simulink model "dqn_C_PQ_HVsMC"  (R2024a)
settings: Solver=FixedStepDiscrete  StartTime=0.0  StopTime=10  FixedStep=Ts_Power  RelTol=1e-3
PreLoadFcn:
  | % HVDCMMCInterconnectionParam
StartFcn:
  | tic
StopFcn:
  | toc
values from neighbouring files (symbols this model uses):
  C_PM = 1.758e-3    (= 0.001758)    [dqnMMCsingle.m]
  Fnom = 50    [dqnMMCsingle.m]
  HRM = 1    [dqnMMCsingle.m]
  Ki_Ireg = 6    [dqnMMCsingle.m]
  Ki_Qreg = 1.0    (= 1)    [dqnMMCsingle.m]
  Kp_Ireg = 0.6    [dqnMMCsingle.m]
  Kp_Qreg = 0.5/3    (= 0.166666666667)    [dqnMMCsingle.m]
  Larm = Larm_pu*(Zb_ac/(2*pi*Fnom))    [dqnMMCsingle.m]
  Larm_pu = 0.15    [dqnMMCsingle.m]
  Lff = Larm_pu/2    (= 0.075)    [dqnMMCsingle.m]
  Limits_Ireg = [ 2.0  -2.0]    [dqnMMCsingle.m]
  Limits_Qreg = [ 0.25, -0.25 ]    [dqnMMCsingle.m]
  Limits_VDCreg = [ 2.0  -2.0]    [dqnMMCsingle.m]
  Lxfo = 0.12    [dqnMMCsingle.m]
  N = 1    [dqnMMCsingle.m]
  Nb_PM = 36    [dqnMMCsingle.m]
  Pnom = 1000e6    (= 1000000000)    [dqnMMCsingle.m]
  R_startup = 400    [dqnMMCsingle.m]
  Rarm = Rarm_pu*Zb_ac    [dqnMMCsingle.m]
  Rff = Rarm_pu/2    (= 0.00075)    [dqnMMCsingle.m]
  Rxfo = 0.003    [dqnMMCsingle.m]
  Slope_Qref = 0.5    [dqnMMCsingle.m]
  Slope_Vdc_ref = Vnom_dc/5    (= 128000)    [dqnMMCsingle.m]
  Tfault = 9999    [dqnMMCsingle.m]
  Ts = Ts_Control    (= 4e-05)    [dqnMMCsingle.m]
  Ts_Control = 40e-6    (= 4e-05)    [dqnMMCsingle.m]
  Ts_dqn = 2e-5    (= 2e-05)    [dqnMMCsingle.m]
  Ts_Power = 20e-6    (= 2e-05)    [dqnMMCsingle.m]
  Vnom_dc = 640e3    (= 640000)    [dqnMMCsingle.m]
  Vnom_prim = 400e3    (= 400000)    [dqnMMCsingle.m]
  Vnom_sec = 333e3    (= 333000)    [dqnMMCsingle.m]
  Ws = 2*pi*50    (= 314.159265359)    [dqnMMCsingle.m]
undefined symbols (not defined in the file or in its folder): DiscIntNeverNeededParam, Discrete, DQN_Lib, gcbh, Int_DQNc_Mat, Mult_DQNc_Mat, Pcc, S, sps, sps_rtmsupport, spsMeanValueVariableFrequencyModel, spsPLL3phModel, SY3
libraries: simulink x18, spsControlledVoltageSourceLib x15, spsVoltageMeasurementLib x9, powerlib_extras x6, spsSecondOrderFilterLib x6, spsCurrentMeasurementLib x6, spsIdealSwitchLib x6, spsMeanLib x4, spsdq0toabcLib x4, spsMeanVariableFrequencyLib x4, spsabctodq0Lib x4, spsThreePhaseSeriesRLCBranchLib x4
(part 1 of 6)
settings Model: SimulationMode=accelerator  Creator=The MathWorks, Inc.  LastModifiedBy=salsarayreh
settings SolverCC: AlgebraicLoopSolver=TrustRegion
settings DataIOCC: SaveFormat=StructureWithTime  SaveOutput=off  DSMLogging=off  SaveTime=off  ReturnWorkspaceOutputs=off
settings OptimizationCC: ReuseModelBlockBuffer=off  ExpressionDepthLimit=2147483647  LifeSpan=inf
settings DebuggingCC: UnderspecifiedInitializationDetection=Classic  MergeDetectMultiDrivingBlocksExec=none  SolverPrmCheckMsg=warning  FcnCallInpInsideContextMsg=warning  UnconnectedInputMsg=warning  UnconnectedOutputMsg=warning  UnconnectedLineMsg=warning  AllowSymbolicDim=off  StateNameClashWarn=warning  SFUnexpectedBacktrackingDiag=warning  SFNoUnconditionalDefaultTransitionDiag=warning  SFExecutionAtInitializationDiag=none  ArithmeticOperatorsInVariantConditions=warning
settings HardwareCC: ProdBitPerPointer=32  ProdBitPerSizeT=32  ProdBitPerPtrDiffT=32  ProdLargestAtomicFloat=None  ProdIntDivRoundTo=Undefined  ProdEndianess=Unspecified  ProdWordSize=32  ProdHWDeviceType=32-bit Generic
settings ModelReferenceCC: EnableRefExpFcnMdlSchedulingChecks=on  PropagateSignalLabelsOutOfModel=off
settings SFSimCC: SimUseLocalCustomCode=off  CustomCodeUndefinedFunction=UseInterfaceOnly
settings RTWCC: RTWUseLocalCustomCode=off  GPUComputeCapability=3.5
settings CodeAppCC: StateflowObjectComments=on
settings GRTTargetCC: TargetLangStandard=C89/C90 (ANSI)  CombineOutputUpdateFcns=off  GRTInterface=on
settings ConfigComp: CovMetricSettings=dw  CovSaveCumulativeToWorkspaceVar=on  CovSaveSingleToWorkspaceVar=on  CovExternalEMLEnable=off
settings SimscapeCC: SimscapeNormalizeSystem=off

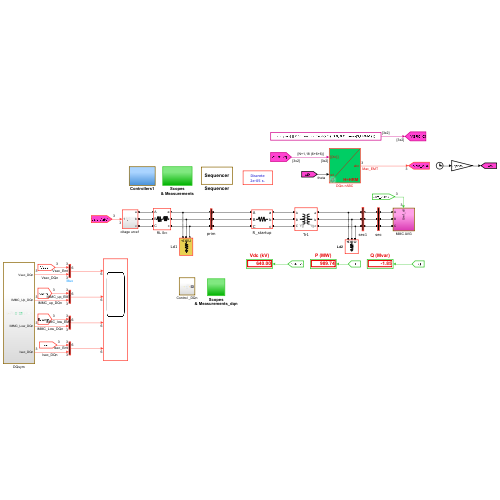
[thumbnail: Simulink's stored preview of the top-level diagram]
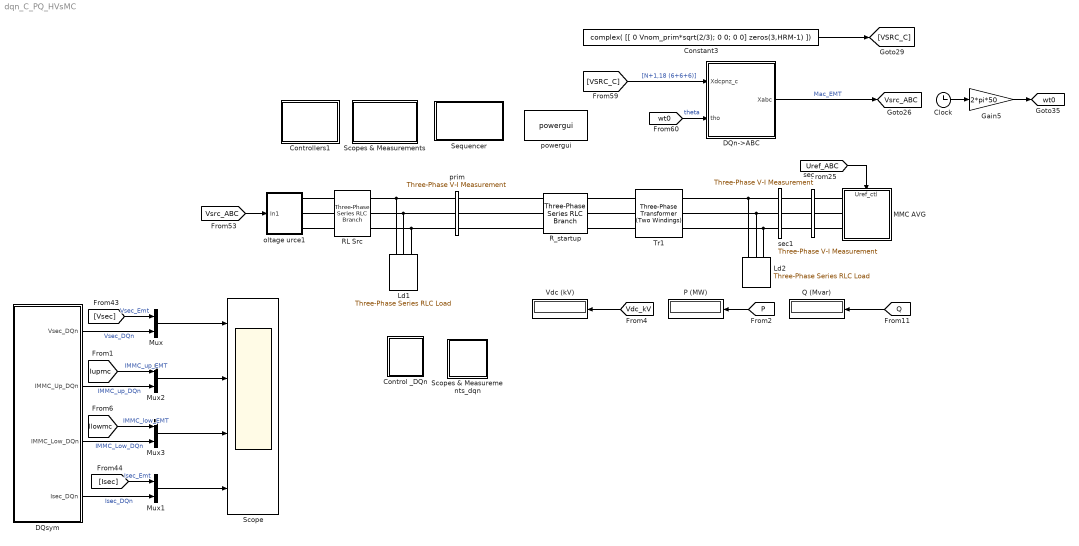
== system dqn_C_PQ_HVsMC ==
  Clock : Clock
  Constant3 : Constant  Value=complex( [[ 0 Vnom_prim*sqrt(2/3); 0 0; 0 0] zeros(3,HRM-1) ])
  Control _DQn : Subsystem
  Controllers1 : Subsystem
  DQn->ABC : MATLAB Function  TreatAsAtomicUnit=on  SystemSampleTime=Ts_Power  mask{N=HRM}
      mask prompts: N "Harmonic order:"
  DQsym : Subsystem
  Gain5 : Gain  Gain=2*pi*50
  Ld1 : spsThreePhaseSeriesRLCLoadLib/Three-Phase Series RLC Load  LConnTagsString=A|B|C  Configuration=Y (grounded)  NominalVoltage=Vnom_prim  Vabc=[1e3 1e3 1e3]  Vabcp=[1e3 1e3 1e3]  NominalFrequency=Fnom  UnbalancedPower=off  ActivePower=P_Ld1  InductivePower=0  CapacitivePower=0  Pabc=[10e3 9e3 11e3]  QLabc=[100 90 110]  QCabc=[100 90 110]  Pabcp=[10e3 9e3 11e3]  QLabcp=[100 90 110]  QCabcp=[100 90 110]  Measurements=None  LoadType=constant Z
  Ld2 : spsThreePhaseSeriesRLCLoadLib/Three-Phase Series RLC Load  LConnTagsString=A|B|C  Configuration=Y (grounded)  NominalVoltage=Vnom_sec  Vabc=[1e3 1e3 1e3]  Vabcp=[1e3 1e3 1e3]  NominalFrequency=Fnom  UnbalancedPower=off  ActivePower=500e3  InductivePower=0  CapacitivePower=0  Pabc=[10e3 9e3 11e3]  QLabc=[100 90 110]  QCabc=[100 90 110]  Pabcp=[10e3 9e3 11e3]  QLabcp=[100 90 110]  QCabcp=[100 90 110]  Measurements=None  LoadType=constant Z
  MMC AVG : Subsystem
      settings: PortSchema="{\"entries\":[{\"content\":{\"sides\":[{\"content\":{\"connectorIds\":[\"LConn1\",\"LConn2\",\"LConn3\"]},\"type\":\"ConnectorPlacement.EquallySpacedRectSide\",\"uuid\":\"ba64873c-b22b-410d-af4d-7ba2fdc55c23\"},{\"content\":{\"side\":\"RIGHT\"},\"type\":\"ConnectorPlacement.EquallySpacedRectSide\",\"uuid\":\"193af711-64d0-4e3f-b9d8-3af97f0f6abc\"},{\"content\":{\"connectorIds\":[\"In1\"],\"side\":\"TOP\"},\"type\":\"ConnectorPlacement.EquallySpacedRectSide\",\"uuid\":\"04826a8d-a462-403d-873f-6ac7e8481113\"}]},\"type\":\"ConnectorPlacement.EquallySpacedConnector\",\"uuid\":\"1def47fd-2da9-40af-b501-c2103dcb1fab\"}],\"packageUris\":[\"http://schema.mathworks.com/mf0/Connector/R2020b\"],\"version\":\"1.0\"}"
  Mux{,1..3} (4 alike) : Mux  Inputs=2
  P (MW) : Display
      settings: Format=bank  Decimation=5000
  Q (Mvar) : Display
      settings: Format=bank  Decimation=5000
  RL Src : spsThreePhaseSeriesRLCBranchLib/Three-Phase Series RLC Branch  LConnTagsString=A|B|C  RConnTagsString=A|B|C  BranchType=RL  Resistance=0.8929  Inductance=16.58e-3  Capacitance=1e-6  Measurements=None
  R_startup : spsThreePhaseSeriesRLCBranchLib/Three-Phase Series RLC Branch  LConnTagsString=A|B|C  RConnTagsString=A|B|C  BranchType=R  Resistance=R_startup/5  Inductance=Vnom_prim^2 / Pcc / (2*pi*Fnom)  Capacitance=1e-6  Measurements=None
  Scope : Scope  NumInputPorts=4
  Scopes & Measurements : Subsystem
  Scopes & Measurements_dqn : Subsystem
  Sequencer : Subsystem
      mask Display: disp('Sequencer')
  Tr1 : spsThreePhaseTransformerTwoWindingsLib/Three-Phase Transformer (Two Windings)  Winding1Connection=Yg  Winding2Connection=Yg  CoreType=Three single-phase transformers  SetSaturation=off  Hysteresis=off  DataFile='hysteresis'  SetInitialFlux=off  Measurements=None  UNITS=pu  NominalPower=[ Pnom , Fnom ]  Winding1="[ Vnom_prim , Rxfo/2,  Lxfo/2 ]"  Winding2="[ Vnom_sec , Rxfo/2,  Lxfo/2 ]"  Rm=1000  Lm=1000  L0=0.5  Saturation=[ 0,0 ; 0.0024,1.2 ; 1.0,1.52 ]  InitialFluxes=[ 0.8 , -0.8 , 0.7 ]  BreakLoop=off  DiscreteSolver=Trapezoidal iterative  DataType=off  TransfoNumber=1
  Vdc (kV) : Display
      settings: Format=bank  Decimation=5000
  oltage urce1 : Subsystem
  powergui : spspowerguiLib/powergui  Priority=1  SimulationMode=Discrete  SampleTime=Ts_Power  frequency=60  Iterations=50  frequencyindice=0  Pbase=100e6  ErrMax=1e-4  UnitsV=kV  UnitsW=MW  buscounter=0  FunctionMessages=off  echomessages=off  EnableUseOfTLC=off  CurrentSourceSwitches=off  DisableSnubberDevices=off  DisableRonSwitches=off  DisableVfSwitches=off  DisplayEquations=off  AutomaticDiscreteSolvers=off  SolverType=Tustin/Backward Euler (TBE)  Interpol=off  ExternalGateDelay=off  methode=off  Ts=10  x0status=blocks  SPID=off  SwTol=0  HookPort=off  NonlinearTolerance=1e-4  nMaxIteration=100  ContinueOnMaxIteration=off  RestoreLinks=warning  ResistiveCurrentMeasurement=off  Frange=[0:2:500]  Ylog=off  Xlog=on  ShowGrid=off  save=off  variable=ZData  structure=VIprim  ZoomFFT=on  StartTime=0.15  cycles=2  DisplayStyle=1  fundamental=50  FreqAxis=on  MaxFrequency=1000  frequencyindicesteady=1  RmsSteady=1  display=off
  prim : spsThreePhaseVIMeasurementLib/Three-Phase V-I Measurement  VoltageMeasurement=phase-to-ground  SetLabelV=on  LabelV=Vprim  Vpu=off  VpuLL=off  CurrentMeasurement=yes  SetLabelI=on  LabelI=Iprim  Ipu=off  Pbase=100e6  Vbase=500e3  OutputType=Complex  PhasorSimulation=off  PSBequivalent=0
  sec : spsThreePhaseVIMeasurementLib/Three-Phase V-I Measurement  VoltageMeasurement=phase-to-ground  SetLabelV=on  LabelV=Vsec  Vpu=off  VpuLL=off  CurrentMeasurement=yes  SetLabelI=on  LabelI=Isec  Ipu=off  Pbase=100e6  Vbase=500e3  OutputType=Complex  PhasorSimulation=off  PSBequivalent=0
  sec1 : spsThreePhaseVIMeasurementLib/Three-Phase V-I Measurement  VoltageMeasurement=no  SetLabelV=on  LabelV=Vsec  Vpu=off  VpuLL=off  CurrentMeasurement=yes  SetLabelI=on  LabelI=Isec2  Ipu=off  Pbase=100e6  Vbase=500e3  OutputType=Complex  PhasorSimulation=off  PSBequivalent=0
  tag scope: Vsrc_ABC=global, wt0=global
  wires:
  [P] -> P (MW)/1
  [Vdc_kV] -> Vdc (kV)/1
  [Q] -> Q (Mvar)/1
  [Uref_ABC] -> MMC AVG/1(Uref_ctl)
  Clock/1 -> Gain5/1
  Gain5/1 -> [wt0]
  [Vsrc_ABC] -> oltage urce1/1(In1)
  DQn->ABC/1(Xabc) -> [Vsrc_ABC]  "Mac_EMT"
  [wt0] -> DQn->ABC/2(tho)  "theta"
  Constant3/1 -> [VSRC_C]
  [VSRC_C] -> DQn->ABC/1(Xdcpnz_c)  "[N+1,18 (6+6+6)]"
  DQsym/1(Vsec_DQn) -> Mux/2  "Vsec_DQn"
  DQsym/4(Isec_DQn) -> Mux1/2  "Isec_DQn"
  DQsym/2(IMMC_Up_DQn) -> Mux2/2  "IMMC_up_DQn"
  DQsym/3(IMMC_Low_DQn) -> Mux3/2  "IMMC_Low_DQn"
  Mux/1 -> Scope/1
  Mux2/1 -> Scope/2
  Mux3/1 -> Scope/3
  Mux1/1 -> Scope/4
  [Vsec] -> Mux/1  "Vsec_Emt"
  [Iupmc] -> Mux2/1  "IMMC_up_EMT"
  [Isec] -> Mux1/1  "Isec_Emt"
  [Ilowmc] -> Mux3/1  "IMMC_low_EMT"
  connections:
  Ld1/LConn1 -- RL Src/RConn1 -- prim/RConn1
  Ld1/LConn2 -- RL Src/RConn2 -- prim/RConn2
  Ld1/LConn3 -- RL Src/RConn3 -- prim/RConn3
  Ld2/LConn1 -- sec1/RConn1 -- Tr1/RConn1
  Ld2/LConn2 -- sec1/RConn2 -- Tr1/RConn2
  Ld2/LConn3 -- sec1/RConn3 -- Tr1/RConn3
  prim/LConn2 -- R_startup/LConn2
  R_startup/RConn1 -- Tr1/LConn1
  R_startup/RConn2 -- Tr1/LConn2
  R_startup/RConn3 -- Tr1/LConn3
  prim/LConn1 -- R_startup/LConn1
  R_startup/LConn3 -- prim/LConn3
  MMC AVG/LConn1 -- sec/LConn1
  MMC AVG/LConn2 -- sec/LConn2
  MMC AVG/LConn3 -- sec/LConn3
  sec1/LConn1 -- sec/RConn1
  sec/RConn2 -- sec1/LConn2
  sec1/LConn3 -- sec/RConn3
  RL Src/LConn1 -- oltage urce1/RConn1
  RL Src/LConn2 -- oltage urce1/RConn2
  RL Src/LConn3 -- oltage urce1/RConn3

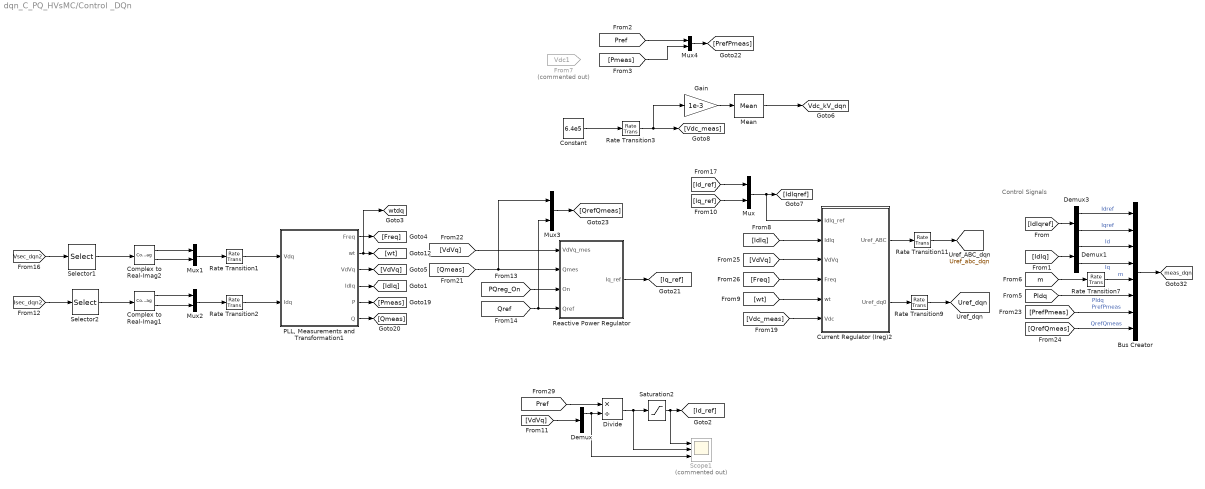
== system dqn_C_PQ_HVsMC/Control _DQn ==
  note: Control Signals
  Bus Creator : BusCreator  Inputs=8
  Complex to Real-Imag1 : ComplexToRealImag
  Complex to Real-Imag2 : ComplexToRealImag
  Constant : Constant  Value=6.4e5
  Current Regulator (Ireg)2 : Subsystem
  Demux : Demux  Outputs=2
  Demux1 : Demux  Outputs=2
  Demux3 : Demux  Outputs=2
  Divide : Product  Inputs=*/
  From7 : From  Commented=on  GotoTag=Vdc1  TagVisibility=global
  Gain : Gain  Gain=1e-3
  Mean : spsMeanLib/Mean  Freq=Fnom/3  Vinit=0  Ts=Ts_Control
  Mux{,1..4} (5 alike) : Mux  Inputs=2
  "PLL, Measurements and Transformation1" : Subsystem
  Rate Transition{1..3,7} (4 alike) : RateTransition  OutPortSampleTime=Ts_Control
  Rate Transition11 : RateTransition  OutPortSampleTime=Ts_Power
  Rate Transition9 : RateTransition  OutPortSampleTime=Ts_Power
  Reactive Power Regulator : Subsystem
  Saturation2 : Saturate  UpperLimit=Limits_VDCreg(1)  LowerLimit=Limits_VDCreg(2)  SampleTime=Ts
  Scope1 : Scope  Commented=on  NumInputPorts=3
  Selector1 : Selector  NumberOfDimensions=2  InputPortWidth=3  IndexOptions=Index vector (dialog),Index vector (dialog)  Indices=1,2  OutputSizes=1,1
  Selector2 : Selector  NumberOfDimensions=2  InputPortWidth=3  IndexOptions=Index vector (dialog),Index vector (dialog)  Indices=1,2  OutputSizes=1,1
  tag scope: Uref_abc_dqn=global, Uref_dqn=global, Vdc_kV_dqn=global, meas_dqn=global, wtdq=global
  wires:
  Complex to Real-Imag2/1 -> Mux1/1
  [PQreg_On] -> Reactive Power Regulator/3(On)
  Selector1/1 -> Complex to Real-Imag2/1
  Complex to Real-Imag2/2 -> Mux1/2
  [Vsec_dqn2] -> Selector1/1
  [Qref] -> Mux3/2, Reactive Power Regulator/4(Qref)
  Complex to Real-Imag1/2 -> Mux2/2
  Selector2/1 -> Complex to Real-Imag1/1
  Complex to Real-Imag1/1 -> Mux2/1
  [Isec_dqn2] -> Selector2/1
  Current Regulator (Ireg)2/1(Uref_ABC) -> Rate Transition11/1
  Mux1/1 -> Rate Transition1/1
  Mux2/1 -> Rate Transition2/1
  Rate Transition1/1 -> "PLL, Measurements and Transformation1"/1(Vdq)
  Rate Transition2/1 -> "PLL, Measurements and Transformation1"/2(Idq)
  Rate Transition11/1 -> [Uref_abc_dqn]
  [PrefPmeas] -> Bus Creator/7  "PrefPmeas"
  [Pref] -> Mux4/1
  [QrefQmeas] -> Bus Creator/8  "QrefQmeas"
  Mux4/1 -> [PrefPmeas]
  Gain/1 -> Mean/1
  [Pmeas] -> Mux4/2
  [m] -> Rate Transition7/1
  Rate Transition3/1 -> Gain/1, [Vdc_meas]
  Demux3/1 -> Bus Creator/1  "Idref"
  Rate Transition7/1 -> Bus Creator/5  "m"
  [IdIq] -> Demux1/1
  Bus Creator/1 -> [meas_dqn]
  Demux1/1 -> Bus Creator/3  "Id"
  Demux3/2 -> Bus Creator/2  "Iqref"
  [IdIqref] -> Demux3/1
  [PIdq] -> Bus Creator/6  "PIdq"
  [Id_ref] -> Mux/1
  Demux1/2 -> Bus Creator/4  "Iq"
  Constant/1 -> Rate Transition3/1
  [Iq_ref] -> Mux/2
  Mean/1 -> [Vdc_kV_dqn]
  "PLL, Measurements and Transformation1"/6(Q) -> [Qmeas]
  "PLL, Measurements and Transformation1"/5(P) -> [Pmeas]
  "PLL, Measurements and Transformation1"/4(IdIq) -> [IdIq]
  "PLL, Measurements and Transformation1"/3(VdVq) -> [VdVq]
  "PLL, Measurements and Transformation1"/2(wt) -> [wtdq], [wt]
  "PLL, Measurements and Transformation1"/1(Freq) -> [Freq]
  Reactive Power Regulator/1(Iq_ref) -> [Iq_ref]
  [Qmeas] -> Mux3/1, Reactive Power Regulator/2(Qmes)
  [VdVq] -> Reactive Power Regulator/1(VdVq_mes)
  Mux3/1 -> [QrefQmeas]
  Mux/1 -> Current Regulator (Ireg)2/1(IdIq_ref), [IdIqref]
  [IdIq] -> Current Regulator (Ireg)2/2(IdIq)
  [VdVq] -> Current Regulator (Ireg)2/3(VdVq)
  [wt] -> Current Regulator (Ireg)2/5(wt)
  [Freq] -> Current Regulator (Ireg)2/4(Freq)
  [Vdc_meas] -> Current Regulator (Ireg)2/6(Vdc)
  Current Regulator (Ireg)2/2(Uref_dq0) -> Rate Transition9/1
  Rate Transition9/1 -> [Uref_dqn]
  Demux/1 -> Scope1/3, Divide/2
  Saturation2/1 -> Scope1/1, [Id_ref]
  Divide/1 -> Scope1/2, Saturation2/1
  [Pref] -> Divide/1
  [VdVq] -> Demux/1

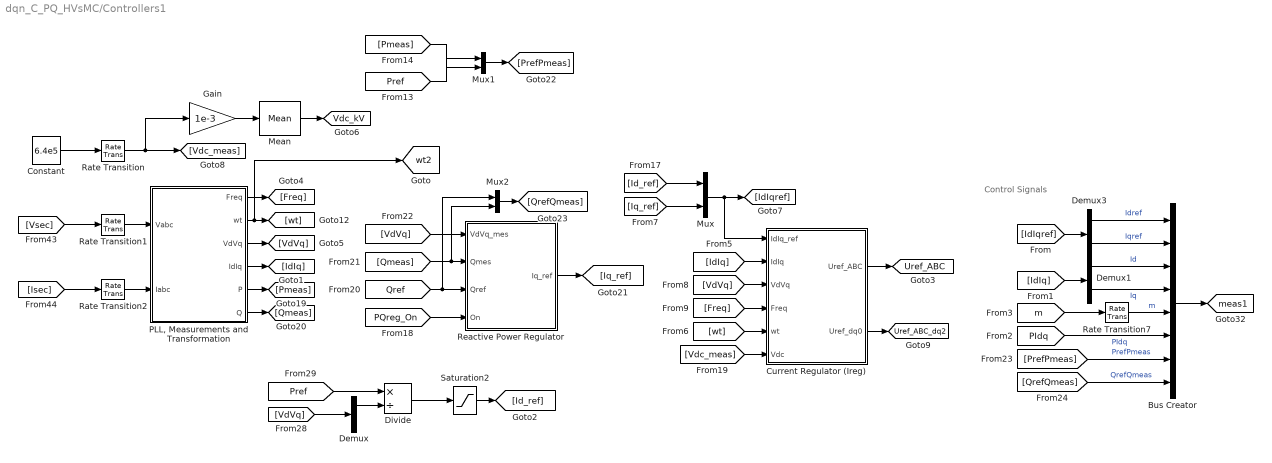
== system dqn_C_PQ_HVsMC/Controllers1 ==
  note: Control Signals
  Bus Creator : BusCreator  Inputs=8
  Constant : Constant  Value=6.4e5
  Current Regulator (Ireg) : Subsystem
  Demux : Demux  Outputs=2
  Demux1 : Demux  Outputs=2
  Demux3 : Demux  Outputs=2
  Divide : Product  Inputs=*/
  Gain : Gain  Gain=1e-3
  Mean : spsMeanLib/Mean  Freq=Fnom/3  Vinit=0  Ts=Ts_Control
  Mux : Mux  Inputs=2
  Mux1 : Mux  Inputs=2
  Mux2 : Mux  Inputs=2
  "PLL, Measurements and Transformation" : Subsystem
  Rate Transition{,1..2,7} (4 alike) : RateTransition  OutPortSampleTime=Ts_Control
  Reactive Power Regulator : Subsystem
  Saturation2 : Saturate  UpperLimit=Limits_VDCreg(1)  LowerLimit=Limits_VDCreg(2)  SampleTime=Ts
  tag scope: Uref_ABC=global, Uref_ABC_dq2=global, Vdc_kV=global, meas1=global, wt2=global
  wires:
  Mean/1 -> [Vdc_kV]
  [Vsec] -> Rate Transition1/1
  [Isec] -> Rate Transition2/1
  [Vdc_meas] -> Current Regulator (Ireg)/6(Vdc)
  Gain/1 -> Mean/1
  Current Regulator (Ireg)/1(Uref_ABC) -> [Uref_ABC]
  [wt] -> Current Regulator (Ireg)/5(wt)
  Constant/1 -> Rate Transition/1
  "PLL, Measurements and Transformation"/2(wt) -> [wt2], [wt]
  "PLL, Measurements and Transformation"/4(IdIq) -> [IdIq]
  [Freq] -> Current Regulator (Ireg)/4(Freq)
  [Id_ref] -> Mux/1
  "PLL, Measurements and Transformation"/3(VdVq) -> [VdVq]
  Mux/1 -> Current Regulator (Ireg)/1(IdIq_ref), [IdIqref]
  Demux1/2 -> Bus Creator/4  "Iq"
  [IdIq] -> Current Regulator (Ireg)/2(IdIq)
  [IdIqref] -> Demux3/1
  Demux3/1 -> Bus Creator/1  "Idref"
  [IdIq] -> Demux1/1
  Bus Creator/1 -> [meas1]
  Demux3/2 -> Bus Creator/2  "Iqref"
  [m] -> Rate Transition7/1
  Demux1/1 -> Bus Creator/3  "Id"
  [PIdq] -> Bus Creator/6  "PIdq"
  "PLL, Measurements and Transformation"/1(Freq) -> [Freq]
  [VdVq] -> Current Regulator (Ireg)/3(VdVq)
  [Iq_ref] -> Mux/2
  Rate Transition/1 -> Gain/1, [Vdc_meas]
  Rate Transition2/1 -> "PLL, Measurements and Transformation"/2(Iabc)
  Rate Transition7/1 -> Bus Creator/5  "m"
  Rate Transition1/1 -> "PLL, Measurements and Transformation"/1(Vabc)
  [PQreg_On] -> Reactive Power Regulator/4(On)
  Mux2/1 -> [QrefQmeas]
  Mux1/1 -> [PrefPmeas]
  [Qref] -> Mux2/1, Reactive Power Regulator/3(Qref)
  [QrefQmeas] -> Bus Creator/8  "QrefQmeas"
  Reactive Power Regulator/1(Iq_ref) -> [Iq_ref]
  "PLL, Measurements and Transformation"/5(P) -> [Pmeas]
  [VdVq] -> Reactive Power Regulator/1(VdVq_mes)
  [Qmeas] -> Mux2/2, Reactive Power Regulator/2(Qmes)
  [Pref] -> Mux1/1
  [PrefPmeas] -> Bus Creator/7  "PrefPmeas"
  "PLL, Measurements and Transformation"/6(Q) -> [Qmeas]
  [Pmeas] -> Mux1/2
  [Pref] -> Divide/1
  Demux/1 -> Divide/2
  Divide/1 -> Saturation2/1
  [VdVq] -> Demux/1
  Saturation2/1 -> [Id_ref]
  Current Regulator (Ireg)/2(Uref_dq0) -> [Uref_ABC_dq2]

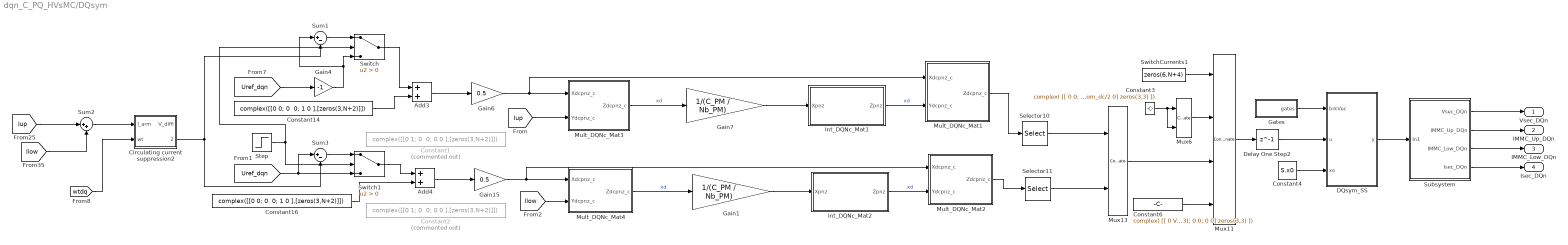
== system dqn_C_PQ_HVsMC/DQsym ==
  Add3 : Sum
  Add4 : Sum
  Circulating current suppression2 : Subsystem  VariantControl=Variant1
  Constant1 : Constant  Commented=on  Value="complex([[0 1; 0  0; 0 0 ],[zeros(3,N+2)]])"
  Constant14 : Constant  Value="complex([[0 0; 0  0; 1 0 ],[zeros(3,N+2)]])"
  Constant16 : Constant  Value="complex([[0 0; 0  0; 1 0 ],[zeros(3,N+2)]])"
  Constant2 : Constant  Commented=on  Value="complex([[0 1; 0  0; 0 0 ],[zeros(3,N+2)]])"
  Constant3 : Constant  Value=complex( [[ 0 0; 0 0; Vnom_dc/2 0] zeros(3,3) ])
  Constant4 : Constant  Value=S.x0  SampleTime=-1
  Constant6 : Constant  Value=complex( [[ 0 Vnom_prim*sqrt(2/3); 0 0; 0 0] zeros(3,3) ])
  DQsym_SS : MATLAB Function  TreatAsAtomicUnit=on  mask{Ad=S.A, Bd=S.B, Cd=S.C, Dd=S.D, swOnRes=1e-3*ones(1,6), swOffRes=1e6*ones(1,6), swType=ones(1,6), InitVec=S.x0, dt=2e-5, nrSWvec=6}
      mask prompts: Ad "A"; Bd "B"; Cd "C"; Dd "D"; swOnRes "Switch on resistance:"; swOffRes "Switch off resistance:"; swType "Switch type:"; InitVec "Initial values:"; dt "Time step (s):"; nrSWvec "Number of switches:"
  Delay One Step2 : Delay  DelayLength=1  SampleTime=2e-5
  Gain1 : Gain  Gain=1/(C_PM / Nb_PM)
  Gain15 : Gain  Gain=0.5
  Gain4 : Gain  Gain=-1
  Gain6 : Gain  Gain=0.5
  Gain7 : Gain  Gain=1/(C_PM / Nb_PM)
  Gates : Subsystem
  Int_DQNc_Mat1 : MATLAB Function  AncestorBlock=DQN_Lib/Int_DQNc_Mat  TreatAsAtomicUnit=on  SystemSampleTime=Ts_dqn  mask{N=8, dt=2e-5, w=Ws, InitInt=0*[0.8; 0.6; -0.33], swFeed=off, R=1, iL=1}
      mask prompts: N "Order number:"; dt "Time step (s):"; w "Angular frequency (1/rad):"; InitInt "Initial conditions DC [3x1]:"; swFeed "Enable feedback"; R "Feedback parameter (Kr {abc}):"; iL "Feedback parameter (Ki {abc}):"
  Int_DQNc_Mat2 : MATLAB Function  AncestorBlock=DQN_Lib/Int_DQNc_Mat  TreatAsAtomicUnit=on  SystemSampleTime=Ts_dqn  mask{N=8, dt=2e-5, w=Ws, InitInt=0*[0.8; 0.6; -0.33], swFeed=off, R=1, iL=1}
      mask prompts: N "Order number:"; dt "Time step (s):"; w "Angular frequency (1/rad):"; InitInt "Initial conditions DC [3x1]:"; swFeed "Enable feedback"; R "Feedback parameter (Kr {abc}):"; iL "Feedback parameter (Ki {abc}):"
  Mult_DQNc_Mat1 : MATLAB Function  AncestorBlock=DQN_Lib/Mult_DQNc_Mat  TreatAsAtomicUnit=on  SystemSampleTime=Ts_dqn  mask{N=8, HrmDbl=on}
      mask prompts: N "Harmonic order:"; HrmDbl "Double Harmonic"
  Mult_DQNc_Mat2 : MATLAB Function  AncestorBlock=DQN_Lib/Mult_DQNc_Mat  TreatAsAtomicUnit=on  SystemSampleTime=Ts_dqn  mask{N=8, HrmDbl=on}
      mask prompts: N "Harmonic order:"; HrmDbl "Double Harmonic"
  Mult_DQNc_Mat3 : MATLAB Function  AncestorBlock=DQN_Lib/Mult_DQNc_Mat  TreatAsAtomicUnit=on  SystemSampleTime=Ts_dqn  mask{N=4, HrmDbl=on}
      mask prompts: N "Harmonic order:"; HrmDbl "Double Harmonic"
  Mult_DQNc_Mat4 : MATLAB Function  AncestorBlock=DQN_Lib/Mult_DQNc_Mat  TreatAsAtomicUnit=on  SystemSampleTime=Ts_dqn  mask{N=4, HrmDbl=on}
      mask prompts: N "Harmonic order:"; HrmDbl "Double Harmonic"
  Mux11 : Concatenate  NumInputs=4  Mode=Multidimensional array
  Mux13 : Concatenate  Mode=Multidimensional array
  Mux6 : Concatenate  Mode=Multidimensional array
  Selector10 : Selector  NumberOfDimensions=2  InputPortWidth=size(SY3.C,1)  IndexOptions=Select all,Index vector (dialog)  Indices=4:6,1:5  OutputSizes=1,1
  Selector11 : Selector  NumberOfDimensions=2  InputPortWidth=size(SY3.C,1)  IndexOptions=Select all,Index vector (dialog)  Indices=4:6,1:5  OutputSizes=1,1
  Step : Step  Time=0.05  SampleTime=0
  Subsystem : Subsystem
  Sum1 : Sum  Inputs=|+-
  Sum2 : Sum  Inputs=|++
  Sum3 : Sum  Inputs=|+-
  Switch : Switch  Criteria=u2 > Threshold  SaturateOnIntegerOverflow=off  InputSameDT=off
  Switch1 : Switch  Criteria=u2 > Threshold  SaturateOnIntegerOverflow=off  InputSameDT=off
  SwitchCurrents1 : Constant  Value=zeros(6,N+4)
  Vsec_DQn : Outport
  IMMC_Up_DQn : Outport  Port=2
  IMMC_Low_DQn : Outport  Port=3
  Isec_DQn : Outport  Port=4
  wires:
  Delay One Step2/1 -> DQsym_SS/2(u)
  Int_DQNc_Mat2/1(Zpnz) -> Mult_DQNc_Mat2/2(Ydcpnz_c)  "xd"
  Step/1 -> Switch/2, Switch1/2
  Constant16/1 -> Add4/2
  Selector11/1 -> Mux13/2
  Gain4/1 -> Sum1/1, Switch/3
  Subsystem/3(IMMC_Low_DQn) -> IMMC_Low_DQn/1
  [wtdq] -> Circulating current suppression2/2(wt)
  [Iup] -> Sum2/1
  SwitchCurrents1/1 -> Mux11/1
  [Ilow] -> Sum2/2
  Mult_DQNc_Mat3/1(Zdcpnz_c) -> Gain7/1  "xd"
  Subsystem/4(Isec_DQn) -> Isec_DQn/1
  Mux13/1 -> Mux11/3
  [Iup] -> Mult_DQNc_Mat3/2(Ydcpnz_c)
  Gates/1(gates) -> DQsym_SS/1(brkVec)
  Switch/1 -> Add3/1
  Gain15/1 -> Mult_DQNc_Mat2/1(Xdcpnz_c), Mult_DQNc_Mat4/1(Xdcpnz_c)
  Subsystem/2(IMMC_Up_DQn) -> IMMC_Up_DQn/1
  [Ilow] -> Mult_DQNc_Mat4/2(Ydcpnz_c)
  Add3/1 -> Gain6/1
  Sum2/1 -> Circulating current suppression2/1(I_arm)
  [Uref_dqn] -> Switch1/3, Sum3/1
  Sum1/1 -> Switch/1
  Mult_DQNc_Mat4/1(Zdcpnz_c) -> Gain1/1  "xd"
  Constant6/1 -> Mux11/4
  Circulating current suppression2/2(-2Uref_dq0) -> Sum1/2, Sum3/2
  Mux11/1 -> Delay One Step2/1
  Switch1/1 -> Add4/1
  Constant14/1 -> Add3/2
  Mult_DQNc_Mat1/1(Zdcpnz_c) -> Selector10/1
  Add4/1 -> Gain15/1
  Mult_DQNc_Mat2/1(Zdcpnz_c) -> Selector11/1
  Constant3/1 -> Mux6/2, Mux6/1
  Mux6/1 -> Mux11/2
  Gain6/1 -> Mult_DQNc_Mat1/1(Xdcpnz_c), Mult_DQNc_Mat3/1(Xdcpnz_c)
  Sum3/1 -> Switch1/1
  Int_DQNc_Mat1/1(Zpnz) -> Mult_DQNc_Mat1/2(Ydcpnz_c)  "xd"
  [Uref_dqn] -> Gain4/1
  Gain1/1 -> Int_DQNc_Mat2/1(Xpnz)
  DQsym_SS/1(y) -> Subsystem/1(In1)
  Constant4/1 -> DQsym_SS/3(xo)
  Gain7/1 -> Int_DQNc_Mat1/1(Xpnz)
  Selector10/1 -> Mux13/1
  Subsystem/1(Vsec_DQn) -> Vsec_DQn/1

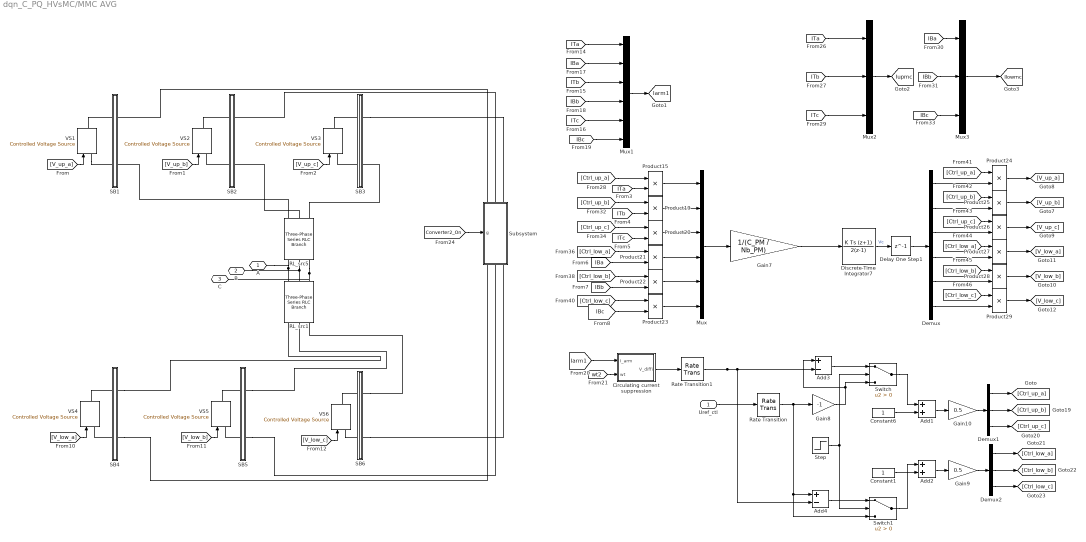
== system dqn_C_PQ_HVsMC/MMC AVG ==
  Uref_ctl : Inport
  Add1 : Sum
  Add2 : Sum
  Add3 : Sum  Inputs=+-
  Add4 : Sum  Inputs=+-
  Circulating current suppression : Subsystem  VariantControl=Variant1
  Constant1 : Constant
  Constant6 : Constant
  Delay One Step1 : Delay  DelayLength=1
  Demux : Demux  Outputs=6
  Demux1 : Demux  Outputs=3
  Demux2 : Demux  Outputs=3
  Discrete-Time Integrator7 : DiscreteIntegrator  IntegratorMethod=Integration: Trapezoidal  gainval=1  SampleTime=Ts_Power  UpperSaturationLimit=5000  LowerSaturationLimit=500  ICPrevOutput=DiscIntNeverNeededParam  ICPrevScaledInput=DiscIntNeverNeededParam
  Gain10 : Gain  Gain=0.5
  Gain7 : Gain  Gain=1/(C_PM / Nb_PM)
  Gain8 : Gain  Gain=-1
  Gain9 : Gain  Gain=0.5
  Mux : Mux  Inputs=6
  Mux1 : Mux  Inputs=6
  Mux2 : Mux  Inputs=3
  Mux3 : Mux  Inputs=3
  Product{15,19..29} (12 alike) : Product
  RL_src1 : spsThreePhaseSeriesRLCBranchLib/Three-Phase Series RLC Branch  LConnTagsString=A|B|C  RConnTagsString=A|B|C  BranchType=RL  Resistance=Rarm  Inductance=Larm  Capacitance=1/(0.55*0.080*(500e3^2/100e6))/(2*pi*60)  Measurements=None
  RL_src5 : spsThreePhaseSeriesRLCBranchLib/Three-Phase Series RLC Branch  LConnTagsString=A|B|C  RConnTagsString=A|B|C  BranchType=RL  Resistance=Rarm  Inductance=Larm  Capacitance=1/(0.55*0.080*(500e3^2/100e6))/(2*pi*60)  Measurements=None
  Rate Transition : RateTransition  OutPortSampleTime=Ts_Power
  Rate Transition1 : RateTransition  OutPortSampleTime=Ts_Power
  SB1 : Subsystem
  SB2 : Subsystem
  SB3 : Subsystem
  SB4 : Subsystem
  SB5 : Subsystem
  SB6 : Subsystem
  Step : Step  SampleTime=0
  Subsystem : Subsystem
      settings: PortSchema="{\"entries\":[{\"content\":{\"sides\":[{\"content\":{\"connectorIds\":[\"In1\"]},\"type\":\"ConnectorPlacement.EquallySpacedRectSide\",\"uuid\":\"6a070030-9d36-4614-a6ed-5c0106204a15\"},{\"content\":{\"side\":\"RIGHT\"},\"type\":\"ConnectorPlacement.EquallySpacedRectSide\",\"uuid\":\"80e8cce1-ebd9-4d3c-9a33-26e83fa71e17\"},{\"content\":{\"connectorIds\":[\"LConn1\",\"LConn2\",\"LConn3\"],\"side\":\"TOP\"},\"type\":\"ConnectorPlacement.EquallySpacedRectSide\",\"uuid\":\"873c34e2-09cd-4b1f-a733-63c02c066783\"},{\"content\":{\"connectorIds\":[\"RConn1\",\"RConn2\",\"RConn3\"],\"side\":\"BOTTOM\"},\"type\":\"ConnectorPlacement.EquallySpacedRectSide\",\"uuid\":\"2e3fd9e5-67ce-4b4a-a343-b8208a9902db\"}]},\"type\":\"ConnectorPlacement.EquallySpacedConnector\",\"uuid\":\"0790a5cd-c0d6-472f-8eb5-e46769681968\"}],\"packageUris\":[\"http://schema.mathworks.com/mf0/Connector/R2020b\"],\"version\":\"1.0\"}"
  Switch : Switch  Criteria=u2 > Threshold  SaturateOnIntegerOverflow=off  InputSameDT=off
  Switch1 : Switch  Criteria=u2 > Threshold  SaturateOnIntegerOverflow=off  InputSameDT=off
  VS{1..6} (6 alike) : spsControlledVoltageSourceLib/Controlled Voltage Source  Initialize=on  Source_Type=AC  Amplitude=0  Phase=0  Frequency=0  Measurements=None
  A : PMIOPort  Side=Left
  B : PMIOPort  Port=2  Side=Left
  C : PMIOPort  Port=3  Side=Left
  tag scope: Iarm1=global, Ilowmc=global, Iupmc=global
  wires:
  Add4/1 -> Switch1/1
  Gain8/1 -> Switch/3, Add3/1
  Add3/1 -> Switch/1
  Rate Transition1/1 -> Add4/2, Add3/2
  [IBa] -> Mux1/2
  Circulating current suppression/1(V_diffi) -> Rate Transition1/1
  Mux1/1 -> [Iarm1]
  [IBc] -> Mux1/6
  [IBb] -> Mux1/4
  Product29/1 -> [V_low_c]
  Constant6/1 -> Add1/2
  Uref_ctl/1 -> Rate Transition/1
  Demux/5 -> Product28/2
  Demux2/2 -> [Ctrl_low_b]
  Product25/1 -> [V_up_b]
  [Ctrl_low_b] -> Product22/1
  Product20/1 -> Mux/3
  Constant1/1 -> Add2/2
  [Ctrl_low_a] -> Product27/1
  Demux1/2 -> [Ctrl_up_b]
  [Ctrl_up_b] -> Product25/1
  Gain9/1 -> Demux2/1
  Demux/6 -> Product29/2
  Gain10/1 -> Demux1/1
  Demux/3 -> Product26/2
  [Ctrl_up_a] -> Product24/1
  Product28/1 -> [V_low_b]
  Demux2/1 -> [Ctrl_low_a]
  [Ctrl_up_c] -> Product26/1
  Product23/1 -> Mux/6
  Demux1/3 -> [Ctrl_up_c]
  Product19/1 -> Mux/2
  [Ctrl_up_c] -> Product20/1
  [Ctrl_low_a] -> Product21/1
  [Ctrl_up_b] -> Product19/1
  [Ctrl_low_c] -> Product23/1
  [Ctrl_up_a] -> Product15/1
  Product27/1 -> [V_low_a]
  Rate Transition/1 -> Gain8/1, Switch1/3, Add4/1
  Discrete-Time Integrator7/1 -> Delay One Step1/1  "Vc"
  Demux/4 -> Product27/2
  Add2/1 -> Gain9/1
  Product21/1 -> Mux/4
  Demux1/1 -> [Ctrl_up_a]
  Step/1 -> Switch/2, Switch1/2
  [ITa] -> Mux1/1
  [ITc] -> Mux1/5
  Product22/1 -> Mux/5
  Mux/1 -> Gain7/1
  Demux2/3 -> [Ctrl_low_c]
  Delay One Step1/1 -> Demux/1
  Product26/1 -> [V_up_c]
  Demux/2 -> Product25/2
  [Ctrl_low_c] -> Product29/1
  Product15/1 -> Mux/1
  [Ctrl_low_b] -> Product28/1
  Product24/1 -> [V_up_a]
  Add1/1 -> Gain10/1
  [wt2] -> Circulating current suppression/2(wt)
  [ITb] -> Mux1/3
  [Iarm1] -> Circulating current suppression/1(I_arm)
  Demux/1 -> Product24/2
  Gain7/1 -> Discrete-Time Integrator7/1
  [V_up_c] -> VS3/1
  [V_low_a] -> VS4/1
  [V_up_a] -> VS1/1
  [V_low_b] -> VS5/1
  [V_up_b] -> VS2/1
  [V_low_c] -> VS6/1
  [ITa] -> Product15/2
  [ITc] -> Product20/2
  [ITb] -> Product19/2
  [IBa] -> Product21/2
  [IBb] -> Product22/2
  [IBc] -> Product23/2
  [Converter2_On] -> Subsystem/1(g)
  [ITb] -> Mux2/2
  [ITc] -> Mux2/3
  [ITa] -> Mux2/1
  Mux2/1 -> [Iupmc]
  [IBa] -> Mux3/1
  [IBb] -> Mux3/2
  [IBc] -> Mux3/3
  Mux3/1 -> [Ilowmc]
  Switch1/1 -> Add2/1
  Switch/1 -> Add1/1
  connections:
  VS1/LConn1 -- SB1/LConn2
  SB5/LConn2 -- VS5/LConn1
  RL_src5/LConn2 -- SB2/RConn2
  SB3/LConn1 -- VS3/RConn1
  SB4/LConn2 -- VS4/LConn1
  SB2/LConn1 -- VS2/RConn1
  SB5/RConn1 -- RL_src1/LConn2
  SB6/LConn1 -- VS6/RConn1
  SB6/RConn1 -- RL_src1/LConn3
  SB4/RConn1 -- RL_src1/LConn1
  VS1/RConn1 -- SB1/LConn1
  SB4/LConn1 -- VS4/RConn1
  RL_src5/LConn3 -- SB3/RConn2
  SB5/LConn1 -- VS5/RConn1
  VS6/LConn1 -- SB6/LConn2
  SB3/LConn2 -- VS3/LConn1
  SB2/LConn2 -- VS2/LConn1
  RL_src1/RConn1 -- A/RConn1 -- RL_src5/RConn1
  RL_src1/RConn2 -- RL_src5/RConn2 -- B/RConn1
  RL_src1/RConn3 -- RL_src5/RConn3 -- C/RConn1
  RL_src5/LConn1 -- SB1/RConn2
  Subsystem/LConn1 -- SB1/RConn1
  Subsystem/LConn2 -- SB2/RConn1
  SB3/RConn1 -- Subsystem/LConn3
  SB4/RConn2 -- Subsystem/RConn1
  SB5/RConn2 -- Subsystem/RConn2
  SB6/RConn2 -- Subsystem/RConn3

== system dqn_C_PQ_HVsMC/Scopes & Measurements ==
  Bus Selector : BusSelector  OutputSignals=Idref,Id,Iqref,Iq
  Bus Selector1 : BusSelector  Commented=on  OutputSignals=m,PIdq
  Bus Selector2 : BusSelector  OutputSignals=PrefPmeas,QrefQmeas
  Demux : Demux  Outputs=2
  Demux1 : Demux  Outputs=2
  Gain3 : Gain  Gain=Pnom*1e-6
  Gain4 : Gain  Gain=Pnom*1e-6
  IdIq : Scope  NumInputPorts=2
  Mux{1..4} (4 alike) : Mux  Inputs=2
  PQmeas_MVA : Scope  NumInputPorts=2
  m  PIdq : Scope  Commented=on  NumInputPorts=2
  tag scope: P=global, Q=global
  wires:
  Gain4/1 -> Demux1/1
  Gain3/1 -> Demux/1
  Mux2/1 -> PQmeas_MVA/2  "Qref Qmeas"
  Bus Selector2/2 -> Gain4/1  "<QrefQmeas>"
  Bus Selector2/1 -> Gain3/1  "<PrefPmeas>"
  Mux1/1 -> PQmeas_MVA/1  "Pref Pmeas"
  [meas1] -> Bus Selector2/1
  Bus Selector/4 -> Mux4/2  "<Iq>"
  Bus Selector/3 -> Mux4/1  "<Iqref>"
  Bus Selector/2 -> Mux3/2  "<Id>"
  Bus Selector/1 -> Mux3/1  "<Idref>"
  Mux4/1 -> IdIq/2  "Iqref  Iq"
  Mux3/1 -> IdIq/1  "Idref  Id"
  Bus Selector1/2 -> m  PIdq/2  "<PIdq>"
  Bus Selector1/1 -> m  PIdq/1  "<m>"
  [meas1] -> Bus Selector/1, Bus Selector1/1
  Demux/1 -> Mux1/1
  Demux/2 -> [P], Mux1/2
  Demux1/1 -> Mux2/1
  Demux1/2 -> [Q], Mux2/2

== system dqn_C_PQ_HVsMC/Scopes & Measurements_dqn ==
  Bus Selector : BusSelector  OutputSignals=Idref,Id,Iqref,Iq
  Bus Selector1 : BusSelector  Commented=on  OutputSignals=m,PIdq
  Bus Selector2 : BusSelector  OutputSignals=PrefPmeas,QrefQmeas
  Demux : Demux  Outputs=2
  Demux1 : Demux  Outputs=2
  Gain3 : Gain  Gain=Pnom*1e-6
  Gain4 : Gain  Gain=Pnom*1e-6
  Goto14 : Goto  Commented=on  GotoTag=P  TagVisibility=global
  Goto2 : Goto  Commented=on  GotoTag=Q  TagVisibility=global
  IdIq : Scope  NumInputPorts=2
  Mux{1..4} (4 alike) : Mux  Inputs=2
  PQmeas_MVA : Scope  NumInputPorts=2
  m  PIdq : Scope  Commented=on  NumInputPorts=2
  wires:
  Demux1/2 -> Mux2/2, Goto2/1
  Demux1/1 -> Mux2/1
  Demux/2 -> Mux1/2, Goto14/1
  Demux/1 -> Mux1/1
  [meas_dqn] -> Bus Selector1/1, Bus Selector/1
  Bus Selector1/1 -> m  PIdq/1  "<m>"
  Bus Selector1/2 -> m  PIdq/2  "<PIdq>"
  Mux3/1 -> IdIq/1  "Idref  Id"
  Mux4/1 -> IdIq/2  "Iqref  Iq"
  Bus Selector/1 -> Mux3/1  "<Idref>"
  Bus Selector/2 -> Mux3/2  "<Id>"
  Bus Selector/3 -> Mux4/1  "<Iqref>"
  Bus Selector/4 -> Mux4/2  "<Iq>"
  [meas_dqn] -> Bus Selector2/1
  Mux1/1 -> PQmeas_MVA/1  "Pref Pmeas"
  Bus Selector2/1 -> Gain3/1  "<PrefPmeas>"
  Bus Selector2/2 -> Gain4/1  "<QrefQmeas>"
  Mux2/1 -> PQmeas_MVA/2  "Qref Qmeas"
  Gain3/1 -> Demux/1
  Gain4/1 -> Demux1/1

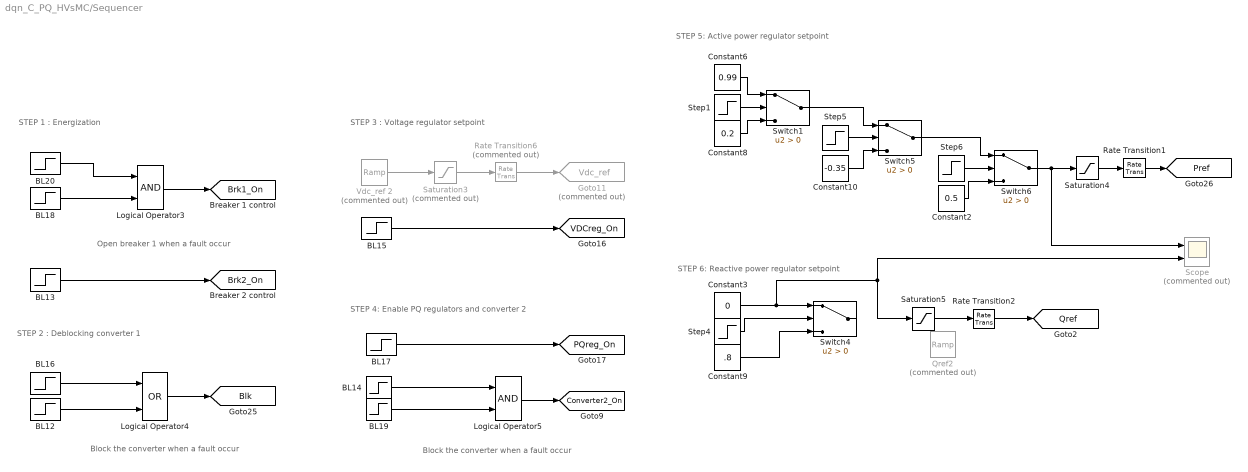
== system dqn_C_PQ_HVsMC/Sequencer ==
  note: STEP 2 : Deblocking converter 1
  note: STEP 6: Reactive power regulator setpoint
  note: STEP 1 : Energization
  note: Block the converter when a fault occur
  note: STEP 5: Active power regulator setpoint
  note: STEP 3 : Voltage regulator setpoint
  note: STEP 4: Enable PQ regulators and converter 2
  note: Block the converter when a fault occur
  note: Open breaker 1 when a fault occur
  BL12 : Step  Time=Tfault+Ts_Power  SampleTime=Ts_Power
  BL13 : Step  Time=0.18  SampleTime=Ts_Power
  BL14 : Step  Time=0.1  SampleTime=Ts_Power
  BL15 : Step  Time=0.07  SampleTime=Ts
  BL16 : Step  Time=0.07  Before=1  After=0  SampleTime=Ts_Power
  BL17 : Step  Time=0.07  SampleTime=Ts
  BL18 : Step  Time=Tfault + 1.95*(1/Fnom)  Before=1  After=0  SampleTime=Ts_Power
  BL19 : Step  Time=Tfault + 2*(1/Fnom)  Before=1  After=0  SampleTime=Ts_Power
  BL20 : Step  Time=0.15  SampleTime=Ts_Power
  Constant10 : Constant  Value=-0.35
  Constant2 : Constant  Value=0.5
  Constant3 : Constant  Value=0
  Constant6 : Constant  Value=0.99
  Constant8 : Constant  Value=0.2
  Constant9 : Constant  Value=.8
  Goto11 : Goto  Commented=on  GotoTag=Vdc_ref  TagVisibility=global
  Logical Operator3 : Logic  AllPortsSameDT=off  OutDataTypeStr=boolean
  Logical Operator4 : Logic  Operator=OR  AllPortsSameDT=off  OutDataTypeStr=float('double')
  Logical Operator5 : Logic  AllPortsSameDT=off  OutDataTypeStr=boolean
  Qref2 : simulink/Sources/Ramp  Commented=on  slope=Slope_Qref  start=Tramping_Qref  InitialOutput=0
  Rate Transition1 : RateTransition  OutPortSampleTime=Ts_Control
  Rate Transition2 : RateTransition  OutPortSampleTime=Ts_Control
  Rate Transition6 : RateTransition  Commented=on  OutPortSampleTime=Ts_Control
  Saturation3 : Saturate  Commented=on  UpperLimit=Vnom_dc  LowerLimit=eps
  Saturation4 : Saturate  UpperLimit=1  LowerLimit=-1
  Saturation5 : Saturate  UpperLimit=Limits_Qreg(1)  LowerLimit=Limits_Qreg(2)
  Scope : Scope  Commented=on  NumInputPorts=2
  Step1 : Step  Time=4  Before=1  After=0  SampleTime=0
  Step4 : Step  Time=3  Before=1  After=0  SampleTime=0
  Step5 : Step  Time=6  Before=1  After=0  SampleTime=0
  Step6 : Step  Time=8  Before=1  After=0  SampleTime=0
  Switch{1,4..6} (4 alike) : Switch  Criteria=u2 > Threshold  SaturateOnIntegerOverflow=off  InputSameDT=off
  Vdc_ref 2 : simulink/Sources/Ramp  Commented=on  slope=Slope_Vdc_ref  start=Tramping_Vdc_ref  InitialOutput=Vnom_sec*1.37
  tag scope: Blk=global, Brk1_On=global, Brk2_On=global, Converter2_On=global, PQreg_On=global, Pref=global, Qref=global, VDCreg_On=global
  wires:
  Constant2/1 -> Switch6/3
  Logical Operator5/1 -> [Converter2_On]
  BL20/1 -> Logical Operator3/1
  Switch6/1 -> Scope/1, Saturation4/1
  Switch5/1 -> Switch6/1
  BL14/1 -> Logical Operator5/1
  Constant3/1 -> Saturation5/1, Scope/2, Switch4/1
  Saturation4/1 -> Rate Transition1/1
  Logical Operator4/1 -> [Blk]
  Switch1/1 -> Switch5/1
  Vdc_ref 2/1 -> Saturation3/1
  Saturation5/1 -> Rate Transition2/1
  BL17/1 -> [PQreg_On]
  BL15/1 -> [VDCreg_On]
  BL18/1 -> Logical Operator3/2
  Logical Operator3/1 -> [Brk1_On]
  Constant6/1 -> Switch1/1
  BL16/1 -> Logical Operator4/1
  BL12/1 -> Logical Operator4/2
  Rate Transition6/1 -> Goto11/1
  Rate Transition1/1 -> [Pref]
  Rate Transition2/1 -> [Qref]
  Step1/1 -> Switch1/2
  Constant9/1 -> Switch4/3
  Step4/1 -> Switch4/2
  Constant8/1 -> Switch1/3
  BL19/1 -> Logical Operator5/2
  Constant10/1 -> Switch5/3
  Saturation3/1 -> Rate Transition6/1
  BL13/1 -> [Brk2_On]
  Step5/1 -> Switch5/2
  Step6/1 -> Switch6/2

== system dqn_C_PQ_HVsMC/oltage urce1 ==
  In1 : Inport
  Demux9 : Demux  Outputs=3
  Ground : spsGroundLib/Ground  LConnTagsString=a
  VSRC_a : spsControlledVoltageSourceLib/Controlled Voltage Source  Initialize=on  Source_Type=AC  Amplitude=0  Phase=0  Frequency=0  Measurements=None
  VSRC_b : spsControlledVoltageSourceLib/Controlled Voltage Source  Initialize=on  Source_Type=AC  Amplitude=0  Phase=0  Frequency=0  Measurements=None
  VSRC_c : spsControlledVoltageSourceLib/Controlled Voltage Source  Initialize=on  Source_Type=AC  Amplitude=0  Phase=0  Frequency=0  Measurements=None
  a : PMIOPort  Side=Right
  b : PMIOPort  Port=2  Side=Right
  c : PMIOPort  Port=3  Side=Right
  wires:
  Demux9/3 -> VSRC_c/1
  Demux9/2 -> VSRC_b/1
  Demux9/1 -> VSRC_a/1
  In1/1 -> Demux9/1
  connections:
  VSRC_a/RConn1 -- a/RConn1
  VSRC_b/RConn1 -- b/RConn1
  VSRC_c/RConn1 -- c/RConn1
  VSRC_c/LConn1 -- VSRC_a/LConn1 -- VSRC_b/LConn1 -- Ground/LConn1

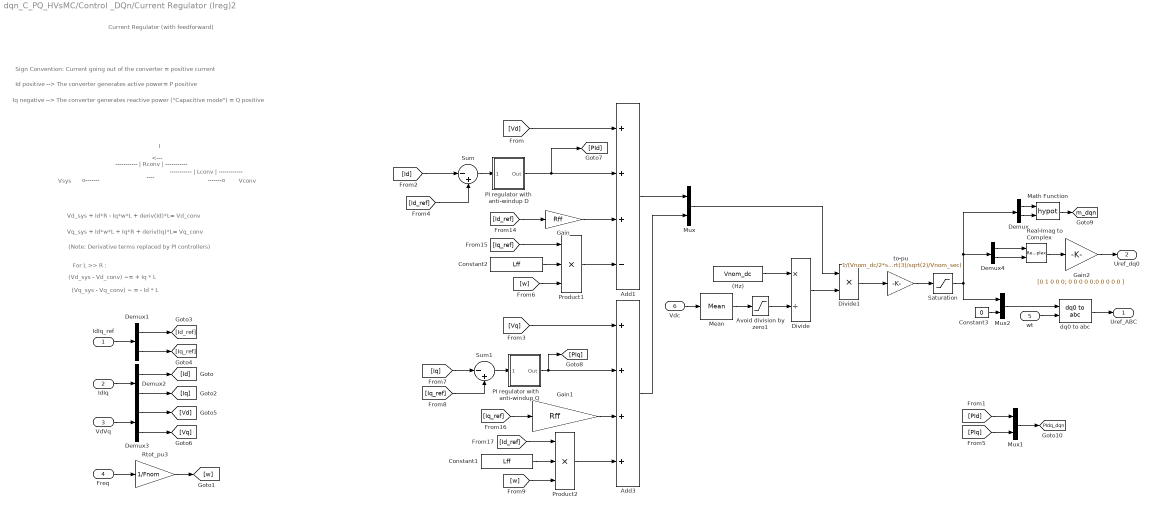
== system dqn_C_PQ_HVsMC/Control _DQn/Current Regulator (Ireg)2 ==
  note: -----------
      | | Lconv |
      | ------------
  note: <---
  note: -------o
  note: Vconv
  note: ----
  note: -----------
      | | Rconv |
      | -----------
  note: For L >> R :
  note: (Vq_sys - Vq_conv) ~ = - Id * L
  note: (Vd_sys - Vd_conv) ~= + Iq * L
  note: Id positive --> The converter generates active power= P positive
  note: Iq negative --> The converter generates reactive power ("Capacitive mode") = Q positive
  note: Sign Convention: Current going out of the converter = positive current
  note: Current Regulator
      | (with feedforward)
  note: Vq_sys + Id*w*L + Iq*R + deriv(Iq)*L= Vq_conv
  note: Vd_sys + Id*R - Iq*w*L + deriv(Id)*L= Vd_conv
  note: (Note: Derivative terms replaced by PI controllers)
  note: Vsys
  note: o-------
  note: I
  IdIq_ref : Inport  PortDimensions=2
  IdIq : Inport  Port=2  PortDimensions=2
  VdVq : Inport  Port=3  PortDimensions=2
  Freq : Inport  Port=4  PortDimensions=1
  wt : Inport  Port=5  PortDimensions=1
  Vdc : Inport  Port=6  PortDimensions=1
  " (Hz)" : Constant  Value=Vnom_dc  SampleTime=Ts
  Add1 : Sum  Inputs=+++-
  Add3 : Sum  Inputs=++++
  Avoid division by zero1 : Saturate  UpperLimit=Vnom_dc*1.25  LowerLimit=Vnom_dc*0.75
  Constant1 : Constant  Value=Lff  SampleTime=Ts_Control
  Constant2 : Constant  Value=Lff  SampleTime=Ts_Control
  Constant3 : Constant  Value=0  SampleTime=Ts
  Demux{,1..4} (5 alike) : Demux  Outputs=2
  Divide : Product  Inputs=*/
  Divide1 : Product  Inputs=**
  Gain : Gain  Gain=Rff
  Gain1 : Gain  Gain=Rff
  Gain2 : Gain  Gain=[0 1 0 0 0; 0 0 0 0 0;0 0 0 0 0 ]
  Math Function : Math  Operator=hypot  SignedPower=on
  Mean : spsMeanLib/Mean  Freq=Fnom/3  Vinit=Vnom_dc  Ts=Ts
  Mux : Mux  Inputs=2
  Mux1 : Mux  Inputs=2
  Mux2 : Mux  Inputs=[2 1]
  PI regulator with anti-windup D : Subsystem  DialogController=POWERSYS.PowerSysDialog  mask(Discrete PI Controller){Kp=Kp_Ireg, Ki=Ki_Ireg, Par_Limits=Limits_Ireg, Init=0, Ts=Ts}
      mask prompts: Kp "Proportional gain (Kp):"; Ki "Integral gain (Ki):"; Par_Limits "Output limits: [ Upper   Lower ]"; Init "Output initial value:"; Ts "Sample time:"
      mask help: This block implements a discrete PI controller.
      mask init:
      | UpperLimit=Par_Limits(1);
      | LowerLimit=Par_Limits(2);
      | power_initmask();
      mask Help: This block is part of a subset of blocks in the Extras library that does not have documentation associated with it, other than the block mask description.
      mask Display: disp('PI');
  PI regulator with anti-windup Q : Subsystem  DialogController=POWERSYS.PowerSysDialog  mask(Discrete PI Controller){Kp=Kp_Ireg, Ki=Ki_Ireg, Par_Limits=Limits_Ireg, Init=0, Ts=Ts}
      mask prompts: Kp "Proportional gain (Kp):"; Ki "Integral gain (Ki):"; Par_Limits "Output limits: [ Upper   Lower ]"; Init "Output initial value:"; Ts "Sample time:"
      mask help: This block implements a discrete PI controller.
      mask init:
      | UpperLimit=Par_Limits(1);
      | LowerLimit=Par_Limits(2);
      | power_initmask();
      mask Help: This block is part of a subset of blocks in the Extras library that does not have documentation associated with it, other than the block mask description.
      mask Display: disp('PI');
  Product1 : Product  Inputs=3  RndMeth=Zero
  Product2 : Product  Inputs=3  RndMeth=Zero
  Real-Imag to Complex : RealImagToComplex
  Rtot_pu3 : Gain  Gain=1/Fnom  SaturateOnIntegerOverflow=on  OutDataTypeStr=Inherit: Same as input  ParamDataTypeStr=Inherit: Same as input
  Saturation : Saturate  UpperLimit=Limits_Ireg(1)  LowerLimit=Limits_Ireg(2)
  Sum : Sum  Inputs=|-+
  Sum1 : Sum  Inputs=|-+
  dq0 to abc : spsdq0toabcLib/dq0 to abc  Alignment=90 degrees behind phase A axis
  to-pu : Gain  Gain=1/(Vnom_dc/2*sqrt(3)/sqrt(2)/Vnom_sec)
  Uref_ABC : Outport
  Uref_dq0 : Outport  Port=2
  tag scope: PIdq_dqn=global, m_dqn=global
  wires:
  to-pu/1 -> Saturation/1
  Mux/1 -> Divide1/1
  dq0 to abc/1 -> Uref_ABC/1
  Divide/1 -> Divide1/2
  Mean/1 -> Avoid division by zero1/1
  Divide1/1 -> to-pu/1
  " (Hz)"/1 -> Divide/1
  Vdc/1 -> Mean/1
  Avoid division by zero1/1 -> Divide/2
  Mux1/1 -> [PIdq_dqn]
  Constant3/1 -> Mux2/2
  Mux2/1 -> dq0 to abc/1
  PI regulator with anti-windup D/1(Out) -> [PId], Add1/2
  PI regulator with anti-windup Q/1(Out) -> [PIq], Add3/2
  [Vd] -> Add1/1
  Product1/1 -> Add1/4
  Gain/1 -> Add1/3
  Gain1/1 -> Add3/3
  Product2/1 -> Add3/4
  [Vq] -> Add3/1
  Demux2/1 -> [Id]
  IdIq/1 -> Demux2/1
  [Id_ref] -> Product2/1
  [Iq_ref] -> Gain1/1
  [Iq_ref] -> Product1/1
  [Id_ref] -> Gain/1
  [Id] -> Sum/1
  [Iq] -> Sum1/1
  Demux2/2 -> [Iq]
  [PIq] -> Mux1/2
  [PId] -> Mux1/1
  [w] -> Product1/3
  Constant2/1 -> Product1/2
  [w] -> Product2/3
  Constant1/1 -> Product2/2
  [Iq_ref] -> Sum1/2
  Sum1/1 -> PI regulator with anti-windup Q/1(Error)
  [Id_ref] -> Sum/2
  Sum/1 -> PI regulator with anti-windup D/1(Error)
  VdVq/1 -> Demux3/1
  Demux3/2 -> [Vq]
  Demux3/1 -> [Vd]
  IdIq_ref/1 -> Demux1/1
  Demux1/2 -> [Iq_ref]
  Demux1/1 -> [Id_ref]
  Rtot_pu3/1 -> [w]
  Freq/1 -> Rtot_pu3/1
  Add1/1 -> Mux/1
  Add3/1 -> Mux/2
  wt/1 -> dq0 to abc/2
  Demux4/2 -> Real-Imag to Complex/2
  Demux4/1 -> Real-Imag to Complex/1
  Real-Imag to Complex/1 -> Gain2/1
  Gain2/1 -> Uref_dq0/1
  Math Function/1 -> [m_dqn]
  Demux/1 -> Math Function/1
  Demux/2 -> Math Function/2
  Saturation/1 -> Demux/1, Demux4/1, Mux2/1

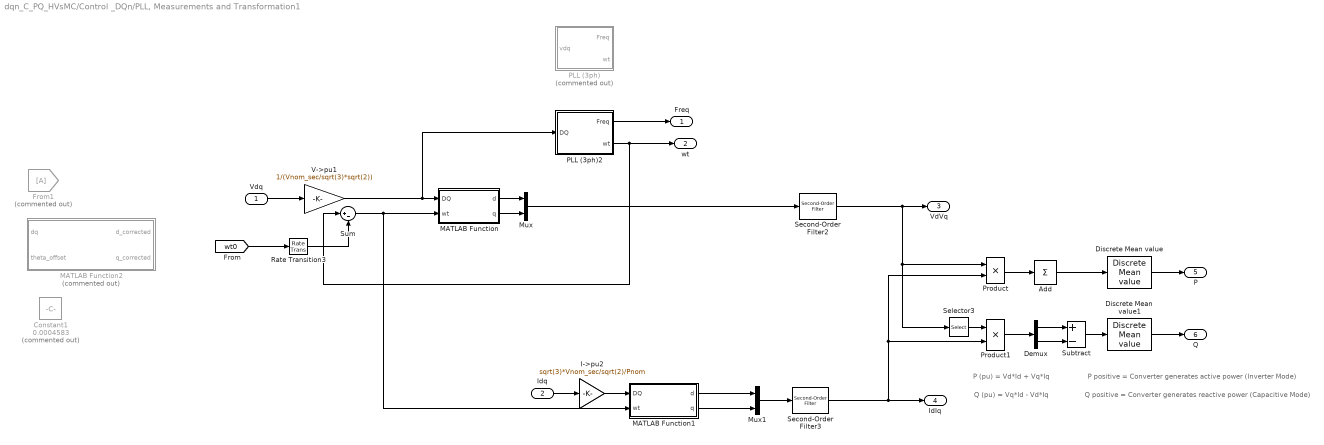
== system dqn_C_PQ_HVsMC/Control _DQn/PLL, Measurements and Transformation1 ==
  note: Q positive = Converter generates reactive power (Capacitive Mode)
  note: P positive = Converter generates active power (Inverter Mode)
  note: Q (pu) = Vq*Id - Vd*Iq
  note: P (pu) = Vd*Id + Vq*Iq
  Vdq : Inport
  Idq : Inport  Port=2
  Add : Sum  Inputs=1
  Constant1 : Constant  Commented=on  Value=0.0004583
  Demux : Demux  Outputs=2
  Discrete Mean value : powerlib_extras/Discrete Measurements/Discrete  Mean value  Freq=Fnom  Vinit=0  Ts=Ts
  Discrete Mean value1 : powerlib_extras/Discrete Measurements/Discrete  Mean value  Freq=Fnom  Vinit=0  Ts=Ts
  From1 : From  Commented=on  TagVisibility=global
  I->pu2 : Gain  Gain=sqrt(3)*Vnom_sec/sqrt(2)/Pnom  SaturateOnIntegerOverflow=on  OutDataTypeStr=Inherit: Same as input  ParamDataTypeStr=Inherit: Same as input
  MATLAB Function : MATLAB Function  TreatAsAtomicUnit=on
  MATLAB Function1 : MATLAB Function  TreatAsAtomicUnit=on
  MATLAB Function2 : MATLAB Function  Commented=on  TreatAsAtomicUnit=on
  Mux : Mux  Inputs=2
  Mux1 : Mux  Inputs=2
  PLL (3ph) : Subsystem  Commented=on  AncestorBlock=|  DialogController=POWERSYS.PowerSysDialog  LoadFcn=sps_rtmsupport('LoadFcn', gcbh);  StartFcn=sps_rtmsupport('StartFcn', gcbh);  StopFcn=sps_rtmsupport('StopFcn', gcbh);  mask(PLL (3ph)){Fmin=0.9*Fnom, Par_Init=[0, Fnom], ParK=[180, 3200, 1], TcD=1e-4, MaxRateChangeFreq=12, FilterCutOffFreq=25, Ts=Ts, AGC=on}
      | spsPLL3phLib/PLL
      | (3ph)
      mask prompts: Fmin "Minimum frequency (Hz):"; Par_Init "Initial inputs [ Phase (degrees), Frequency (Hz) ]:"; ParK "Regulator gains [ Kp, Ki, Kd ]:"; TcD "Time constant for derivative action (s):"; MaxRateChangeFreq "Maximum rate of change of frequency (Hz/s):"; FilterCutOffFreq "Filter cut-off frequency for frequency measurement (Hz):"; Ts "Sample time:"; AGC "Enable automatic gain control"
      mask help:
      | This Phase Locked Loop (PLL) system can be used  to synchronize on a set of variable frequency, three-phase sinusoidal signals. If the Automatic Gain Control is enabled, the input (phase error) of the PLL regulator is scaled according to the input signals magnitude.
      |
      | For optimal performance, set regulator gains [ Kp Ki  Kd ] = [ 180  3200  1 ] and check the Enable Automatic Gain Control parameter.
      |
      | Input : Vector containing the normalized three-phase signals [Va Vb Vc]
      | Output 1:  Measured frequency (Hz) = w/(2pi)
      | Output 2:  Ramp w.t varying between  0 and 2*pi, synchronized on zero crossings of the fundamental (positive-sequence) of phase A.
      mask init:
      | block=gcb;
      | [WantBlockChoice,Ts,sps] = powericon('PLL3phInit',block,Fmin,Par_Init,ParK,TcD, MaxRateChangeFreq, FilterCutOffFreq, AGC,Ts);
      | powericon('SetInternalModels','set',block,WantBlockChoice);
      settings: CopyFcn=sps_rtmsupport('CopyFcn', gcbh);  DeleteFcn=sps_rtmsupport('DeleteFcn', gcbh);  UndoDeleteFcn=sps_rtmsupport('UndoDeleteFcn', gcbh);  ModelCloseFcn=sps_rtmsupport('ModelCloseFcn', gcbh);  PreSaveFcn=sps_rtmsupport('PreSaveFcn', gcbh);  PostSaveFcn=sps_rtmsupport('PostSaveFcn', gcbh);  NameChangeFcn=sps_rtmsupport('NameChangeFcn', gcbh);  PreCopyFcn=sps_rtmsupport('PreCopyFcn', gcbh);  OpenFcn=sps_rtmsupport('OpenFcn', gcbh, [8]);  CloseFcn=sps_rtmsupport('CloseFcn', gcbh);  PreDeleteFcn=sps_rtmsupport('PreDeleteFcn', gcbh);
      mask Help: helpview(psbhelp);
  PLL (3ph)2 : Subsystem  AncestorBlock=|  DialogController=POWERSYS.PowerSysDialog  LoadFcn=sps_rtmsupport('LoadFcn', gcbh);  StartFcn=sps_rtmsupport('StartFcn', gcbh);  StopFcn=sps_rtmsupport('StopFcn', gcbh);  mask(PLL (3ph)){Fmin=0.9*Fnom, Par_Init=[0, Fnom], ParK=[180, 3200, 1], TcD=1e-4, MaxRateChangeFreq=12, FilterCutOffFreq=25, Ts=Ts, AGC=on}
      | spsPLL3phLib/PLL
      | (3ph)
      mask prompts: Fmin "Minimum frequency (Hz):"; Par_Init "Initial inputs [ Phase (degrees), Frequency (Hz) ]:"; ParK "Regulator gains [ Kp, Ki, Kd ]:"; TcD "Time constant for derivative action (s):"; MaxRateChangeFreq "Maximum rate of change of frequency (Hz/s):"; FilterCutOffFreq "Filter cut-off frequency for frequency measurement (Hz):"; Ts "Sample time:"; AGC "Enable automatic gain control"
      mask help:
      | This Phase Locked Loop (PLL) system can be used  to synchronize on a set of variable frequency, three-phase sinusoidal signals. If the Automatic Gain Control is enabled, the input (phase error) of the PLL regulator is scaled according to the input signals magnitude.
      |
      | For optimal performance, set regulator gains [ Kp Ki  Kd ] = [ 180  3200  1 ] and check the Enable Automatic Gain Control parameter.
      |
      | Input : Vector containing the normalized three-phase signals [Va Vb Vc]
      | Output 1:  Measured frequency (Hz) = w/(2pi)
      | Output 2:  Ramp w.t varying between  0 and 2*pi, synchronized on zero crossings of the fundamental (positive-sequence) of phase A.
      mask init:
      | block=gcb;
      | [WantBlockChoice,Ts,sps] = powericon('PLL3phInit',block,Fmin,Par_Init,ParK,TcD, MaxRateChangeFreq, FilterCutOffFreq, AGC,Ts);
      | powericon('SetInternalModels','set',block,WantBlockChoice);
      settings: CopyFcn=sps_rtmsupport('CopyFcn', gcbh);  DeleteFcn=sps_rtmsupport('DeleteFcn', gcbh);  UndoDeleteFcn=sps_rtmsupport('UndoDeleteFcn', gcbh);  ModelCloseFcn=sps_rtmsupport('ModelCloseFcn', gcbh);  PreSaveFcn=sps_rtmsupport('PreSaveFcn', gcbh);  PostSaveFcn=sps_rtmsupport('PostSaveFcn', gcbh);  NameChangeFcn=sps_rtmsupport('NameChangeFcn', gcbh);  PreCopyFcn=sps_rtmsupport('PreCopyFcn', gcbh);  OpenFcn=sps_rtmsupport('OpenFcn', gcbh, [8]);  CloseFcn=sps_rtmsupport('CloseFcn', gcbh);  PreDeleteFcn=sps_rtmsupport('PreDeleteFcn', gcbh);
      mask Help: helpview(psbhelp);
  Product : Product  RndMeth=Zero
  Product1 : Product  RndMeth=Zero
  Rate Transition3 : RateTransition  OutPortSampleTime=Ts_Control
  Second-Order Filter2 : spsSecondOrderFilterLib/Second-Order Filter  FilterType=Lowpass  Fo=Fn_filter  Zeta=Zeta_filter  Ts=Ts  Initialize=off  Vac_Init="[0,  0,  60]"  Vdc_Init=0  PlotResponse=off  FreqRange=[0, 500, 1]
  Second-Order Filter3 : spsSecondOrderFilterLib/Second-Order Filter  FilterType=Lowpass  Fo=Fn_filter  Zeta=Zeta_filter  Ts=Ts  Initialize=off  Vac_Init="[0,  0,  60]"  Vdc_Init=0  PlotResponse=off  FreqRange=[0, 500, 1]
  Selector3 : Selector  InputPortWidth=2  IndexOptions=Index vector (dialog)  Indices=[2 1]  OutputSizes=1
  Subtract : Sum  Inputs=+-
  Sum : Sum  Inputs=|+-
  V->pu1 : Gain  Gain=1/(Vnom_sec/sqrt(3)*sqrt(2))  SaturateOnIntegerOverflow=on  OutDataTypeStr=Inherit: Same as input  ParamDataTypeStr=Inherit: Same as input
  Freq : Outport
  wt : Outport  Port=2
  VdVq : Outport  Port=3
  IdIq : Outport  Port=4
  P : Outport  Port=5
  Q : Outport  Port=6
  wires:
  Idq/1 -> I->pu2/1
  PLL (3ph)2/2(wt) -> Sum/1, wt/1
  Vdq/1 -> V->pu1/1
  PLL (3ph)2/1(Freq) -> Freq/1
  Subtract/1 -> Discrete Mean value1/1
  Add/1 -> Discrete Mean value/1
  Demux/2 -> Subtract/2
  Demux/1 -> Subtract/1
  Product1/1 -> Demux/1
  Product/1 -> Add/1
  Discrete Mean value/1 -> P/1
  Discrete Mean value1/1 -> Q/1
  Selector3/1 -> Product1/1
  Second-Order Filter2/1 -> Selector3/1, Product/1, VdVq/1
  Second-Order Filter3/1 -> Product/2, Product1/2, IdIq/1
  MATLAB Function/1(d) -> Mux/1
  Sum/1 -> MATLAB Function1/2(wt), MATLAB Function/2(wt)
  MATLAB Function/2(q) -> Mux/2
  Mux/1 -> Second-Order Filter2/1
  V->pu1/1 -> PLL (3ph)2/1(DQ), MATLAB Function/1(DQ)
  Mux1/1 -> Second-Order Filter3/1
  MATLAB Function1/1(d) -> Mux1/1
  I->pu2/1 -> MATLAB Function1/1(DQ)
  MATLAB Function1/2(q) -> Mux1/2
  Rate Transition3/1 -> Sum/2
  [wt0] -> Rate Transition3/1
